simulink library "csu_imp_imager_messsage_processing_lib"  (R2014b)
settings: Solver=ode45  StartTime=0.0  StopTime=10.0  RelTol=1e-3
libraries: util_info_lib x1
settings Model: Creator=escrane  LastModifiedBy=mstewart

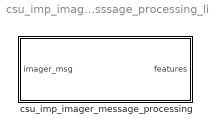
== system csu_imp_imager_messsage_processing_lib ==
  csu_imp_imager_message_processing : Subsystem

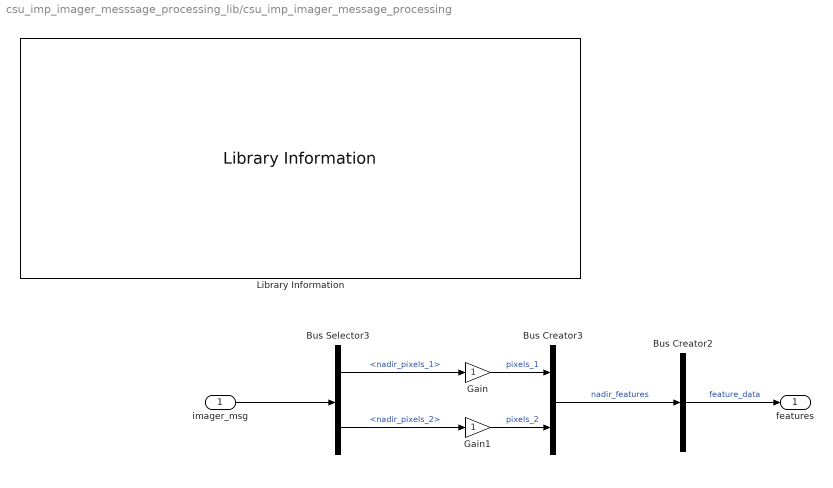
== system csu_imp_imager_messsage_processing_lib/csu_imp_imager_message_processing ==
  imager_msg : Inport
  Bus Creator2 : BusCreator  Inputs=1
  Bus Creator3 : BusCreator  Inputs=2
  Bus Selector3 : BusSelector  OutputSignals=nadir_pixels_1,nadir_pixels_2
  Gain : Gain
  Gain1 : Gain
  Library Information : util_info_lib/Library Information  owner='escrane'
  features : Outport
  wires:
  imager_msg/1 -> Bus Selector3/1
  Bus Creator2/1 -> features/1  "feature_data"
  Bus Selector3/2 -> Gain1/1  "<nadir_pixels_2>"
  Bus Selector3/1 -> Gain/1  "<nadir_pixels_1>"
  Gain/1 -> Bus Creator3/1  "pixels_1"
  Gain1/1 -> Bus Creator3/2  "pixels_2"
  Bus Creator3/1 -> Bus Creator2/1  "nadir_features"
